simulink subsystem "subsys_courant"  (R2021a)
settings: Solver=VariableStepAuto  StartTime=0.0  StopTime=10.0  RelTol=1e-3
settings Model: Creator=antho  LastModifiedBy=alexi

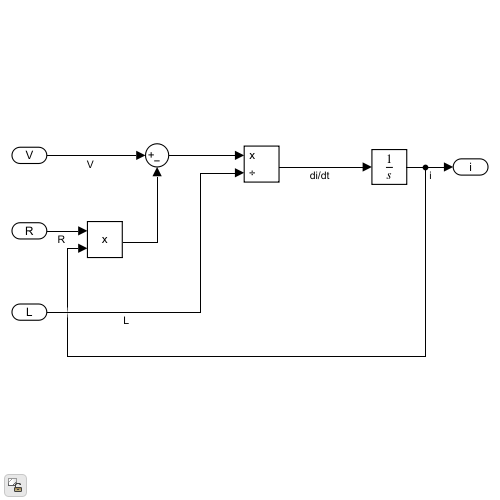
[thumbnail: Simulink's stored preview of the top-level diagram]
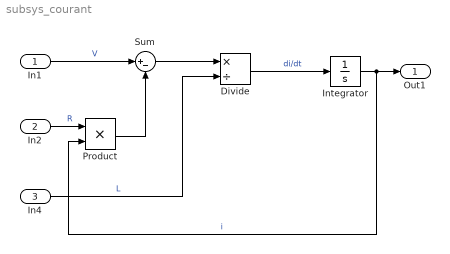
== system subsys_courant ==
  In1 : Inport
  In2 : Inport  Port=2
  In4 : Inport  Port=3
  Divide : Product  Inputs=*/
  Integrator : Integrator
  Product : Product
  Sum : Sum  Inputs=|+-
  Out1 : Outport
  wires:
  In4/1 -> Divide/2  "L"
  In1/1 -> Sum/1  "V"
  Integrator/1 -> Product/2, Out1/1  "i"
  Sum/1 -> Divide/1
  In2/1 -> Product/1  "R"
  Product/1 -> Sum/2
  Divide/1 -> Integrator/1  "di/dt"
